simulink model "model"  (R2022a)
settings: Solver=VariableStepAuto  StartTime=0.0  StopTime=Tf  RelTol=1e-3
undefined symbols (not defined in the file or in its folder): alpha, Atz, Bd, Bh, gama, sigbuilder_block, theta, Ts, Tz_init
libraries: dspsrcs4 x2, rllib x1
settings Model: Creator=masdoua1  LastModifiedBy=masdoua1

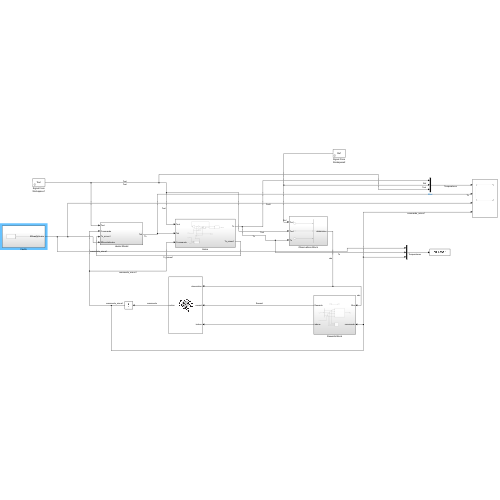
[thumbnail: Simulink's stored preview of the top-level diagram]
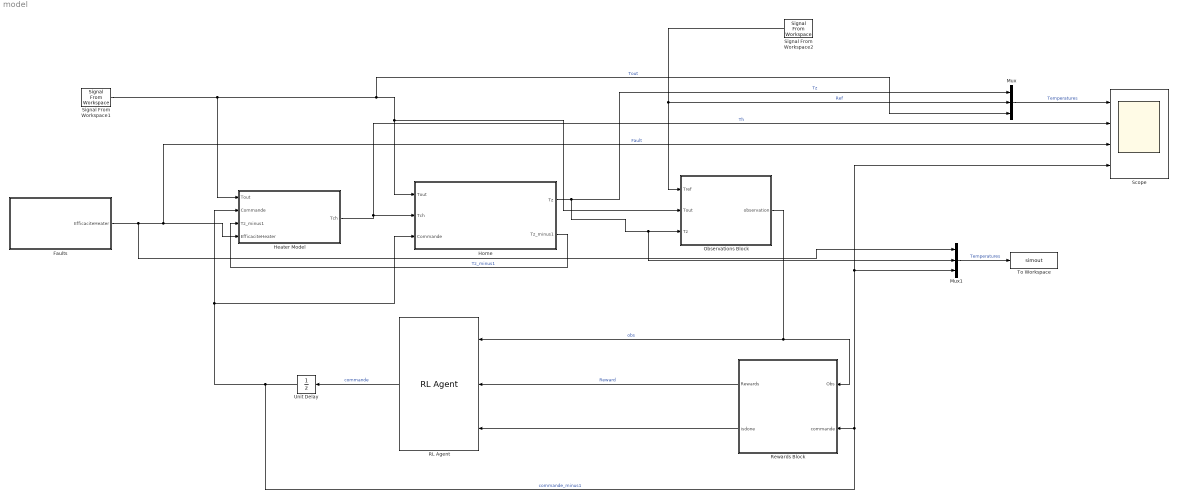
== system model ==
  Faults : Subsystem
  Heater Model : Subsystem
  Home : Subsystem
  Mux : Mux  Inputs=3
  Mux1 : Mux  Inputs=3
  Observations Block : Subsystem
  RL Agent : rllib/RL Agent  Agent=agent  ExternalActionAsInput=off  ProvideLastAction=off  ProvideCumRwd=off  TreatAsDirectFeedthrough=on  UseStrictObservationDataTypes=off
  Rewards Block : Subsystem
  Scope : Scope  NumInputPorts=4
  Signal From Workspace1 : dspsrcs4/Signal From Workspace  X=Tout  Ts=1  nsamps=1  OutputAfterFinalValue=Setting to zero  ignoreOrWarnInputAndFrameLengths=off  OutputFrames=off
  Signal From Workspace2 : dspsrcs4/Signal From Workspace  X=Ref  Ts=1  nsamps=1  OutputAfterFinalValue=Setting to zero  ignoreOrWarnInputAndFrameLengths=off  OutputFrames=off
  To Workspace : ToWorkspace  VariableName=simout  SaveFormat=Timeseries  SampleTime=-1
  Unit Delay : UnitDelay  SampleTime=-1  HasFrameUpgradeWarning=on
  wires:
  Unit Delay/1 -> Rewards Block/2(commande), Mux1/3, Scope/4, Heater Model/2(Commande), Home/3(Commande)  "commande_minus1"
  Signal From Workspace2/1 -> Mux/2, Observations Block/1(Tref)  "Ref"
  Rewards Block/1(Rewards) -> RL Agent/2  "Reward"
  Observations Block/1(observation) -> Rewards Block/1(Obs), RL Agent/1  "obs"
  RL Agent/1 -> Unit Delay/1  "commande"
  Signal From Workspace1/1 -> Heater Model/1(Tout), Observations Block/2(Tout), Home/1(Tout), Mux/3  "Tout"
  Rewards Block/2(isdone) -> RL Agent/3
  Home/1(Tz) -> Mux1/2, Observations Block/3(Tz), Mux/1  "Tz"
  Home/2(Tz_minus1) -> Heater Model/3(Tz_minus1)  "Tz_minus1"
  Heater Model/1(Tch) -> Scope/2, Home/2(Tch)  "Th"
  Mux/1 -> Scope/1  "Temperatures"
  Faults/1(EfficaciteHeater) -> Mux1/1, Scope/3, Heater Model/4(EfficaciteHeater)  "Fault"
  Mux1/1 -> To Workspace/1  "Temperatures"

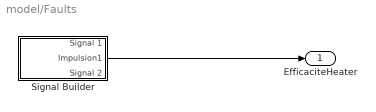
== system model/Faults ==
  Signal Builder : Subsystem  Tag=STV Subsys  LoadFcn=sigbuilder_block('load',[5.4 36 1141.2 516.6 ]);  StartFcn=sigbuilder_block('start');  StopFcn=sigbuilder_block('stop');  ClipboardFcn=sigbuilder_block('clipboard');  mask(Sigbuilder block){tuvar=[0:10]}
      mask help: Simulink:masks:SigbuilderBlock_MD
      mask init:
      | if ~strcmp(get_param(bdroot(gcbh),'SimulationStatus'),'stopped') tuvar = sigbuilder_block('maskInit'); end
      settings: CopyFcn=sigbuilder_block('copy');  DeleteFcn=sigbuilder_block('delete');  ModelCloseFcn=sigbuilder_block('modelClose');  PreSaveFcn=sigbuilder_block('preSave');  PauseFcn=sigbuilder_block('pause');  ContinueFcn=sigbuilder_block('continue');  NameChangeFcn=sigbuilder_block('namechange');  OpenFcn=sigbuilder_block('open',[5.4 36 1141.2 516.6 ]);  CloseFcn=sigbuilder_block('close');
      mask Display: plot(0, 0, 100, 100,[2, 2, 32, 32, 2], [68, 8, 8, 68, 68],[32, 2], [38, 38], [32, 19, 2],[53, 60, 44], [32, 17, 17, 2],[16, 16, 31, 31]);txt = getActiveGroup(gcbh);text(2, 100, txt,'verticalAlignment', 'top');
  EfficaciteHeater : Outport
  wires:
  Signal Builder/2(Impulsion1) -> EfficaciteHeater/1

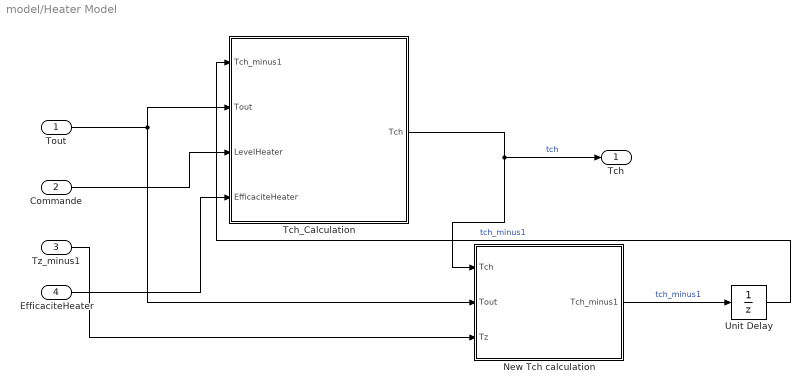
== system model/Heater Model ==
  Tout : Inport
  Commande : Inport  Port=2
  Tz_minus1 : Inport  Port=3
  EfficaciteHeater : Inport  Port=4
  New Tch calculation : Subsystem
  Tch_Calculation : MATLAB Function  TreatAsAtomicUnit=on
  Unit Delay : UnitDelay  SampleTime=-1  HasFrameUpgradeWarning=on
  Tch : Outport
  wires:
  Tout/1 -> New Tch calculation/2(Tout), Tch_Calculation/2(Tout)
  Commande/1 -> Tch_Calculation/3(LevelHeater)
  Tch_Calculation/1(Tch) -> New Tch calculation/1(Tch), Tch/1  "tch"
  Unit Delay/1 -> Tch_Calculation/1(Tch_minus1)  "tch_minus1"
  Tz_minus1/1 -> New Tch calculation/3(Tz)
  New Tch calculation/1(Tch_minus1) -> Unit Delay/1  "tch_minus1"
  EfficaciteHeater/1 -> Tch_Calculation/4(EfficaciteHeater)

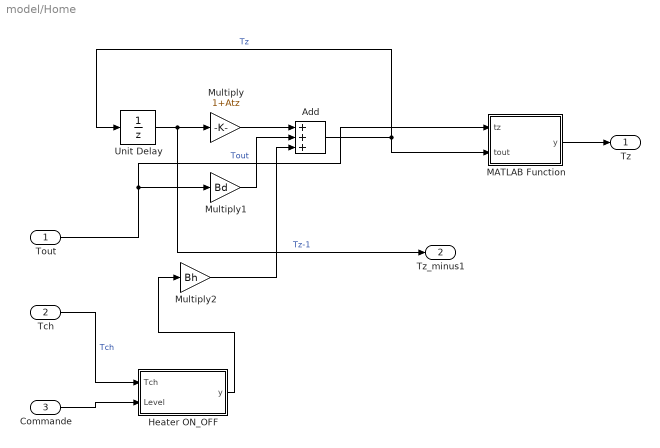
== system model/Home ==
  Tout : Inport
  Tch : Inport  Port=2
  Commande : Inport  Port=3
  Add : Sum  Inputs=+++
  Heater ON_OFF : MATLAB Function  TreatAsAtomicUnit=on
  MATLAB Function : MATLAB Function  TreatAsAtomicUnit=on
  Multiply : Gain  Gain=1+Atz
  Multiply1 : Gain  Gain=Bd
  Multiply2 : Gain  Gain=Bh
  Unit Delay : UnitDelay  InitialCondition=Tz_init  SampleTime=Ts  HasFrameUpgradeWarning=on
  Tz : Outport
  Tz_minus1 : Outport  Port=2
  wires:
  Multiply/1 -> Add/1
  Unit Delay/1 -> Tz_minus1/1, Multiply/1  "Tz-1"
  Tout/1 -> MATLAB Function/1(tz), Multiply1/1  "Tout"
  Multiply1/1 -> Add/2
  Add/1 -> Unit Delay/1, MATLAB Function/2(tout)  "Tz"
  Multiply2/1 -> Add/3
  Commande/1 -> Heater ON_OFF/2(Level)
  Tch/1 -> Heater ON_OFF/1(Tch)  "Tch"
  Heater ON_OFF/1(y) -> Multiply2/1
  MATLAB Function/1(y) -> Tz/1

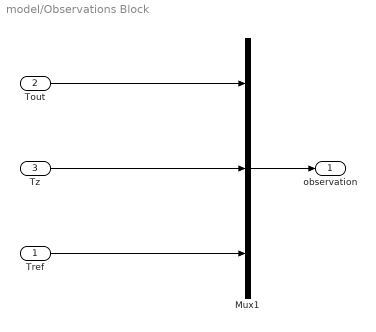
== system model/Observations Block ==
  Tref : Inport
  Tout : Inport  Port=2
  Tz : Inport  Port=3
  Mux1 : Mux  Inputs=3
  observation : Outport
  wires:
  Mux1/1 -> observation/1
  Tz/1 -> Mux1/2
  Tout/1 -> Mux1/1
  Tref/1 -> Mux1/3

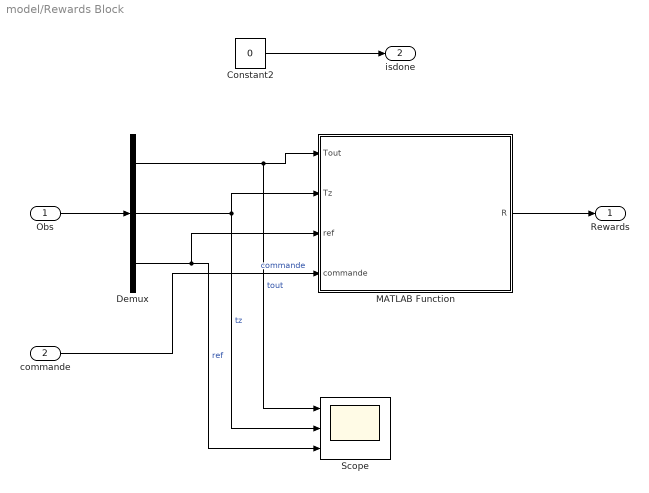
== system model/Rewards Block ==
  Obs : Inport
  commande : Inport  Port=2
  Constant2 : Constant  Value=0
  Demux : Demux  Outputs=3
  MATLAB Function : MATLAB Function  TreatAsAtomicUnit=on
  Scope : Scope  NumInputPorts=3
  Rewards : Outport  VectorParamsAs1DForOutWhenUnconnected=off
  isdone : Outport  Port=2  VectorParamsAs1DForOutWhenUnconnected=off
  wires:
  Constant2/1 -> isdone/1
  MATLAB Function/1(R) -> Rewards/1
  Obs/1 -> Demux/1
  Demux/1 -> Scope/1, MATLAB Function/1(Tout)  "tout"
  Demux/2 -> MATLAB Function/2(Tz), Scope/2  "tz"
  Demux/3 -> MATLAB Function/3(ref), Scope/3  "ref"
  commande/1 -> MATLAB Function/4(commande)  "commande"

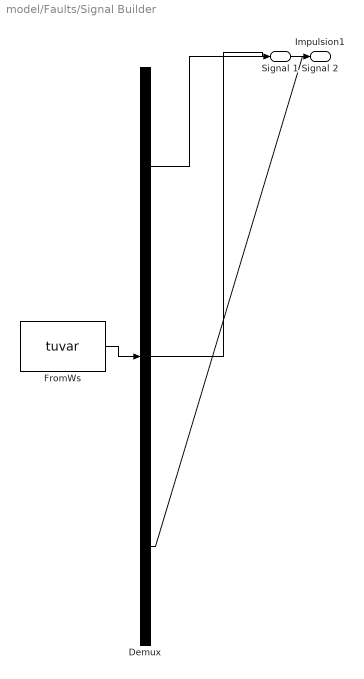
== system model/Faults/Signal Builder ==
  Demux : Demux  Tag=STV Demux  Outputs=3
      settings: DisplayOption=none
  FromWs : FromWorkspace  Tag=STV FromWs  VariableName=tuvar
      SigBuilderData=|
      | common.afterFinalStr = 'Extrapolate'
      | common.sampleTime = 0
      | dataSet.timeRange = [0 24]
      | dataSet.name = 'Group 1'
      | sbobj.Groups.Name = 'Group 1'
      | sbobj.Groups.Signals(1).Name = 'Signal 1'
      | sbobj.Groups.Signals(1).XData = [0 8 8 24]
      | sbobj.Groups.Signals(1).YData = [1 1 0.85 0.85]
      | sbobj.Groups.Signals(2).Name = 'Impulsion1'
      | sbobj.Groups.Signals(2).XData = [0 5 5 6 6 24]
      | sbobj.Groups.Signals(2).YData = [1 1 0.65 0.65 1 1]
      | sbobj.Groups.Signals(3).Name = 'Signal 2'
      | sbobj.Groups.Signals(3).XData = [0 24]
      | sbobj.Groups.Signals(3).YData = [1 1]
      | sbobj.Groups.TimeRange = [0 24]
  Signal 1 : Outport  Tag=STV Outport
  Impulsion1 : Outport  Tag=STV Outport  Port=2
  Signal 2 : Outport  Tag=STV Outport  Port=3
  wires:
  FromWs/1 -> Demux/1
  Demux/1 -> Signal 1/1
  Demux/2 -> Impulsion1/1
  Demux/3 -> Signal 2/1

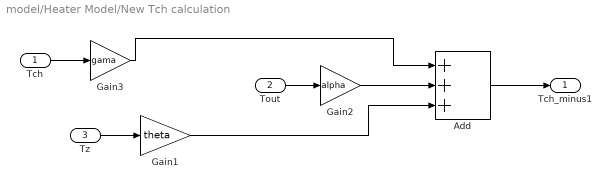
== system model/Heater Model/New Tch calculation ==
  Tch : Inport
  Tout : Inport  Port=2
  Tz : Inport  Port=3
  Add : Sum  Inputs=+++
  Gain1 : Gain  Gain=theta
  Gain2 : Gain  Gain=alpha
  Gain3 : Gain  Gain=gama
  Tch_minus1 : Outport
  wires:
  Add/1 -> Tch_minus1/1
  Gain1/1 -> Add/3
  Tz/1 -> Gain1/1
  Tout/1 -> Gain2/1
  Gain2/1 -> Add/2
  Tch/1 -> Gain3/1
  Gain3/1 -> Add/1

== matlab function model/Heater Model/Tch_Calculation ==
  data: Tch_minus1 input; Tout input; LevelHeater input; Tch output; EfficaciteHeater input
function Tch = fcn(Tch_minus1, Tout, LevelHeater, EfficaciteHeater)
    
    if Tout > Tch_minus1
        Tch_minus1 = Tout+0.2; 
    end
    
    Tch = Tch_minus1 + LevelHeater;
    Tch = Tch*EfficaciteHeater;

== matlab function model/Rewards Block/MATLAB Function ==
  data: Tout input; R output; Tz input; ref input; commande input
function R = fcn(Tout,Tz, ref, commande)

R1 = 0; R2 = 0; R3 = 0;

err = abs(ref - Tz);

% if err <= 0.1
%     R1 = 100;
% elseif err <= 2
%     R1 = 50;
% elseif err <= 4
%     R1 = 10;
% elseif err <= 6
%     R1 = -10;
% else
%     R1 = -100;
% end

% err = abs(Tz-ref);

% if err == 0
%     R1 = 100;
% else
%     R1 = 10*(1/err);
% end

% R1 = - 100 * err;

%% Regulation => erreur = 0.
R1 = -1 * err;

if (err < 1)
    R2 = 2;
end
%% Minimisation energie => Minimisation (Commande)
% R2 = -10 * commande;

R = R1 + R2 + R3;

== matlab function model/Home/Heater ON_OFF ==
  data: Tch input; Level input; y output
function y = fcn(Tch, Level)
y = Tch;
if Level ==0
        y = 0;
end

== matlab function model/Home/MATLAB Function ==
  data: tz input; tout input; y output
function y = fcn(tz, tout)
y = tz;
    if tz < tout
        y = tout;
    end
